simulink model "slxcases_R2021a"  (R2021a)
settings: Solver=VariableStepAuto  StartTime=0.0  StopTime=10.0  RelTol=1e-3
model workspace (MAT data in the model file):
  cfg.mode = 'fast'
  cfg.gain = 2
  flag = 1
  grid = [1  2  3; 4  5  6]
  inner = 7
  label = 'hello'
  names = {'alpha', 'beta'}
  span = 3
  tau = 0.25
undefined symbols (not defined in the file or in its folder): Ki, Kp
settings Model: DataDictionary=slxparams.sldd  Creator=weiwang  LastModifiedBy=weiwang
settings DebuggingCC: UnconnectedInputMsg=none  UnconnectedOutputMsg=none  UnconnectedLineMsg=none
settings ModelReferenceCC: UpdateModelReferenceTargets=IfOutOfDate  EnableRefExpFcnMdlSchedulingChecks=off
settings SFSimCC: SimGPUStackLimitPerThread=51200
settings RTWCC: Description=Generic Real-Time Target  GPUStackLimitPerThread=51200  GPUComputeCapability=7.5  DLArmComputeVersion=20.02.1
settings ConfigComp: CovMetricSettings=de  CovBoundaryAbsTol=1.0e-5

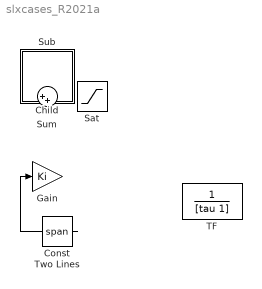
== system slxcases_R2021a ==
  Child : ModelReference  ModelNameDialog=slx_child  ModelReferenceVersion=1.1
  Const : Constant  Value=Kp
  Gain : Gain  Gain=Ki
  Sat : Saturate  UpperLimit=Inf  LowerLimit=-Inf
  Sub : Subsystem
  Sum : Sum  Inputs=|++
  TF : TransferFcn  Denominator=[tau 1]
  Two Lines : Constant  Value=span
  wires:
  Const/1 -> Gain/1

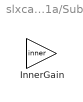
== system slxcases_R2021a/Sub ==
  InnerGain : Gain  Gain=inner
